simulink model "modelSuperLUCbf"  (Simulink 9.2)
settings: Solver=ode45  StartTime=0.0  StopTime=5.0  RelTol=1e-3
values from neighbouring files (symbols this model uses):
  kp1 = w1^2*Mrig(1,1)    [pourDaniel.m]
  kp2 = w2^2*Mrig(2,2)    [pourDaniel.m]
  kv1 = sqrt(2)*w1*Mrig(1,1)    [pourDaniel.m]
  kv2 = sqrt(2)*w2*Mrig(2,2)    [pourDaniel.m]
libraries: cstblocks x1
settings Model: Creator=d.alazard  LastModifiedBy=d.alazard
settings DataIOCC: SignalLoggingSaveFormat=Dataset
settings OptimizationCC: BlockReduction=off  BooleanDataType=off
settings DebuggingCC: SaveWithParameterizedLinksMsg=none  SignalResolutionControl=TryResolveAllWithWarning  FcnCallInpInsideContextMsg=error  AllowSymbolicDim=off  StateNameClashWarn=none
settings HardwareCC: TargetUnknown=on
settings GRTTargetCC: CombineOutputUpdateFcns=on  GRTInterface=off
settings ConfigComp: CovSFcnEnable=off

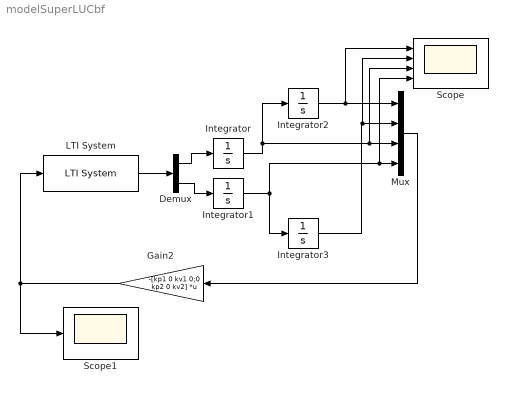
== system modelSuperLUCbf ==
  Demux : Demux  Outputs=2
  Gain2 : Gain  Gain="-[kp1 0 kv1 0;0  kp2 0  kv2]"  Multiplication=Matrix(K*u) (u vector)
  Integrator : Integrator
  Integrator1 : Integrator
  Integrator2 : Integrator
  Integrator3 : Integrator  InitialCondition=10*pi/180
  LTI System : cstblocks/LTI System  sys=Gs  IC=[]
  Mux : Mux
  Scope : Scope  NumInputPorts=4
  Scope1 : Scope
  wires:
  Demux/1 -> Integrator/1
  Demux/2 -> Integrator1/1
  Integrator/1 -> Scope/3, Mux/3, Integrator2/1
  Integrator1/1 -> Integrator3/1, Scope/4, Mux/4
  Integrator2/1 -> Scope/1, Mux/1
  Integrator3/1 -> Scope/2, Mux/2
  Mux/1 -> Gain2/1
  Gain2/1 -> LTI System/1, Scope1/1
  LTI System/1 -> Demux/1
